simulink model "modeltest_model"  (Simulink 8.5)
settings: Solver=ode1  StartTime=0.0  StopTime=0.01  FixedStep=0.01  RelTol=1e-3
undefined symbols (not defined in the file or in its folder): a
settings Model: Creator=nogueira_raf  LastModifiedBy=nogueira_raf
settings DataIOCC: InitialState=2000  SignalLoggingSaveFormat=Dataset  SaveOutput=off  SaveTime=off
settings OptimizationCC: BooleanDataType=off  ExpressionDepthLimit=128
settings DebuggingCC: UnderspecifiedInitializationDetection=Simplified  MergeDetectMultiDrivingBlocksExec=error  FcnCallInpInsideContextMsg=EnableAllAsError  StateNameClashWarn=none
settings GRTTargetCC: CombineOutputUpdateFcns=on  GRTInterface=off

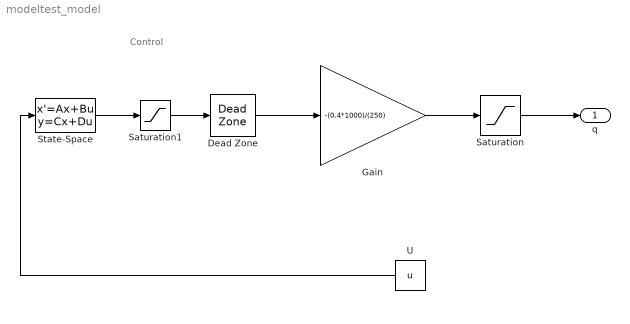
== system modeltest_model ==
  note: Control
  Dead Zone : DeadZone  LowerValue=19250  UpperValue=20750  SaturateOnIntegerOverflow=on
  Gain : Gain  Gain=-(0.4*1000)/(250)
  Saturation : Saturate  UpperLimit=0.4*1000  LowerLimit=-0.4*1000
  Saturation1 : Saturate  UpperLimit=21000  LowerLimit=18000
  State-Space : StateSpace  A=-1/a  B=1/a  D=0  X0=20000
  U : Constant  Value=u
  q : Outport
  wires:
  Gain/1 -> Saturation/1
  Dead Zone/1 -> Gain/1
  Saturation1/1 -> Dead Zone/1
  State-Space/1 -> Saturation1/1
  U/1 -> State-Space/1
  Saturation/1 -> q/1
